simulink model "LINE_CONTROL"  (R2024a)
settings: Solver=ode4  StartTime=0.0  StopTime=10  FixedStep=1e-1  RelTol=1e-3
PreLoadFcn:
  | track_map = track_map;
values from neighbouring files (symbols this model uses):
  D_left = 1    [LINE_CONTROL_SETUP.m]    (also in x_opt.mat = 0.0771620798353)
  D_right = 1    [LINE_CONTROL_SETUP.m]    (also in x_opt.mat = 2.23648591389)
  I_left = 1    [LINE_CONTROL_SETUP.m]    (also in x_opt.mat = 1.054302631)
  I_right = 1    [LINE_CONTROL_SETUP.m]    (also in x_opt.mat = 1.261021045)
  L = 10e-2    (= 0.1)    [LINE_CONTROL_SETUP.m]    (also in x_opt.mat)
  P_left = 1    [LINE_CONTROL_SETUP.m]    (also in x_opt.mat = 2.23919550421)
  P_right = 1    [LINE_CONTROL_SETUP.m]    (also in x_opt.mat = 4.57741332247)
  r = 3.5e-2    (= 0.035)    [LINE_CONTROL_SETUP.m]    (also in x_opt.mat)
  theta_0 = deg2rad(0)    [LINE_CONTROL_SETUP.m]    (also in x_opt.mat = 0)
  x0 = 1    [LINE_CONTROL_SETUP.m]    (also in x_opt.mat)
  y0 = 1.146    [LINE_CONTROL_SETUP.m]    (also in x_opt.mat)
undefined symbols (not defined in the file or in its folder): k_1, k_2, k_3
libraries: slpidlib x2
settings Model: ParamWorkspaceSource=ReferencedWorkspace  Creator=pedro  LastModifiedBy=pedro

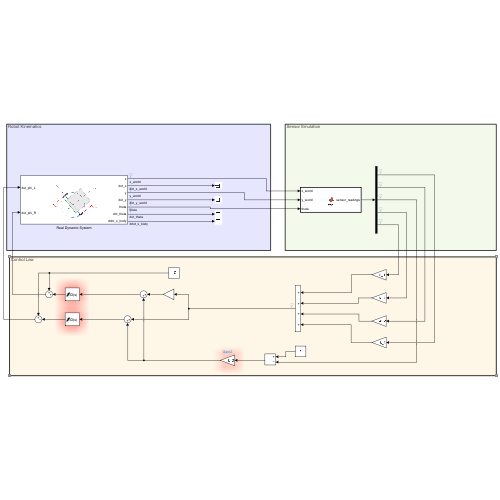
[thumbnail: Simulink's stored preview of the top-level diagram]
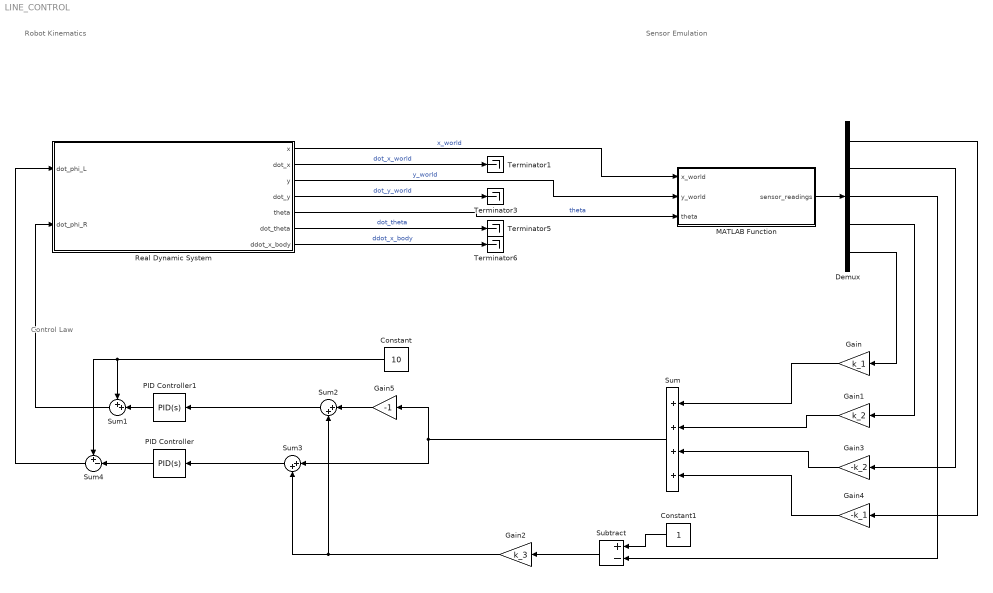
== system LINE_CONTROL ==
  note: Control Law
  note: Sensor Emulation
  note: Robot Kinematics
  Constant : Constant  Value=10
  Constant1 : Constant
  Demux : Demux  Outputs=5
  Gain : Gain  Gain=k_1
  Gain1 : Gain  Gain=k_2
  Gain2 : Gain  Gain=k_3
  Gain3 : Gain  Gain=-k_2
  Gain4 : Gain  Gain=-k_1
  Gain5 : Gain  Gain=-1
  MATLAB Function : MATLAB Function  TreatAsAtomicUnit=on
  PID Controller : slpidlib/PID Controller  Controller=PID  Form=Ideal  TimeDomain=Continuous-time  UseExternalTs=off  SampleTime=-1  IntegratorMethod=Forward Euler  FilterMethod=Forward Euler  ControllerParametersSource=internal  P=P_left  I=I_left  UseKiTs=off  D=D_left  UseExternalDerivativeSource=off  N=100  UseFilter=on  TunerSelectOption=Transfer Function Based (PID Tuner App)  InitialConditionSource=internal  InitialConditionForIntegrator=0  InitialConditionForFilter=0  DifferentiatorICPrevScaledInput=0  ExternalReset=none  TrackingMode=off  Kt=1  LimitOutput=on  SatLimitsSource=internal  UpperSaturationLimit=20  LowerSaturationLimit=-20  LinearizeAsGain=on  AntiWindupMode=clamping  Kb=1  LimitIntegrator=off  UpperIntegratorSaturationLimit=inf  LowerIntegratorSaturationLimit=-inf  POutMin=[]  POutMax=[]  IOutMin=[]  IOutMax=[]  DOutMin=[]  DOutMax=[]  NOutMin=[]  NOutMax=[]  SumOutMin=[]  SumOutMax=[]  SaturationOutMin=[]  SaturationOutMax=[]  PParamMin=[]  PParamMax=[]  IParamMin=[]  IParamMax=[]  DParamMin=[]  DParamMax=[]  NParamMin=[]  NParamMax=[]  KbParamMin=[]  KbParamMax=[]  KtParamMin=[]  KtParamMax=[]  KbOutMin=[]  KbOutMax=[]  KtOutMin=[]  KtOutMax=[]  IntegratorOutMin=[]  IntegratorOutMax=[]  FilterOutMin=[]  FilterOutMax=[]  SumI1OutMin=[]  SumI1OutMax=[]  SumI2OutMin=[]  SumI2OutMax=[]  SumI3OutMin=[]  SumI3OutMax=[]  SumI4OutMin=[]  SumI4OutMax=[]  SumDOutMin=[]  SumDOutMax=[]  DifferentiatorOutMin=[]  DifferentiatorOutMax=[]  FilterDiffOutCoefMin=[]  FilterDiffOutCoefMax=[]  ReciprocalOutMin=[]  ReciprocalOutMax=[]  SumDenOutMin=[]  SumDenOutMax=[]  SumNumOutMin=[]  SumNumOutMax=[]  DivideOutMin=[]  DivideOutMax=[]  UdiffTsProdOutMin=[]  UdiffTsProdOutMax=[]  NTsProdOutMin=[]  NTsProdOutMax=[]  UintegralTsProdOutMin=[]  UintegralTsProdOutMax=[]  UngainTsProdOutMin=[]  UngainTsProdOutMax=[]  ClampingZeroOutDataTypeStr=Inherit: Inherit via back propagation  ClampingZeroOutMin=[]  ClampingZeroOutMax=[]  FilterDenConstantOutDataTypeStr=Inherit: Inherit via back propagation  FilterDenConstantOutMin=[]  FilterDenConstantOutMax=[]  PCopyOutDataTypeStr=Inherit: Inherit via back propagation  PCopyOutMin=[]  PCopyOutMax=[]  NCopyOutDataTypeStr=Inherit: Inherit via back propagation  NCopyOutMin=[]  NCopyOutMax=[]  IntegratorContinuousStateAttributes=''  IntegratorStateMustResolveToSignalObject=off  IntegratorRTWStateStorageClass=Auto  FilterContinuousStateAttributes=''  FilterStateMustResolveToSignalObject=off  FilterRTWStateStorageClass=Auto  ParallelPVariant=Passthrough  IdealPVariant=InternalParameters  IVariant=InternalParameters  DVariant=InternalParameters  IntegratorVariant=Continuous  SatVariant=Enabled  AWVariant=ContClampingIdeal  PCopyVariant=InternalParamsIdeal  TRVariant=Disabled  FdbkBlocksVariant=Forward  IdealPFdbkVariant=Disabled  SatFdbkVariant=Disabled  DerivativeFilterVariant=ContFilter  NVariant=InternalParameters  NCopyVariant=Disabled  FilterICVariant=InternalICsFilter  IntegratorICVariant=InternalICs  ExternalResetVariant=Disabled  TRSumVariant=Passthrough  SumFdbkVariant=Disabled  SumVariant=Sum_PID  TsampFilterVariant=InternalTs  TsampNgainVariant=Passthrough  TsampIntegralVariant=Disabled_SignalSpec  ExternalSaturationOutDataTypeStr=Inherit: Same as second input  DerivativeSourceVariant=ErrorSignal
  PID Controller1 : slpidlib/PID Controller  Controller=PID  Form=Ideal  TimeDomain=Continuous-time  UseExternalTs=off  SampleTime=-1  IntegratorMethod=Forward Euler  FilterMethod=Forward Euler  ControllerParametersSource=internal  P=P_right  I=I_right  UseKiTs=off  D=D_right  UseExternalDerivativeSource=off  N=100  UseFilter=on  TunerSelectOption=Transfer Function Based (PID Tuner App)  InitialConditionSource=internal  InitialConditionForIntegrator=0  InitialConditionForFilter=0  DifferentiatorICPrevScaledInput=0  ExternalReset=none  TrackingMode=off  Kt=1  LimitOutput=on  SatLimitsSource=internal  UpperSaturationLimit=20  LowerSaturationLimit=-20  LinearizeAsGain=on  AntiWindupMode=clamping  Kb=1  LimitIntegrator=off  UpperIntegratorSaturationLimit=inf  LowerIntegratorSaturationLimit=-inf  POutMin=[]  POutMax=[]  IOutMin=[]  IOutMax=[]  DOutMin=[]  DOutMax=[]  NOutMin=[]  NOutMax=[]  SumOutMin=[]  SumOutMax=[]  SaturationOutMin=[]  SaturationOutMax=[]  PParamMin=[]  PParamMax=[]  IParamMin=[]  IParamMax=[]  DParamMin=[]  DParamMax=[]  NParamMin=[]  NParamMax=[]  KbParamMin=[]  KbParamMax=[]  KtParamMin=[]  KtParamMax=[]  KbOutMin=[]  KbOutMax=[]  KtOutMin=[]  KtOutMax=[]  IntegratorOutMin=[]  IntegratorOutMax=[]  FilterOutMin=[]  FilterOutMax=[]  SumI1OutMin=[]  SumI1OutMax=[]  SumI2OutMin=[]  SumI2OutMax=[]  SumI3OutMin=[]  SumI3OutMax=[]  SumI4OutMin=[]  SumI4OutMax=[]  SumDOutMin=[]  SumDOutMax=[]  DifferentiatorOutMin=[]  DifferentiatorOutMax=[]  FilterDiffOutCoefMin=[]  FilterDiffOutCoefMax=[]  ReciprocalOutMin=[]  ReciprocalOutMax=[]  SumDenOutMin=[]  SumDenOutMax=[]  SumNumOutMin=[]  SumNumOutMax=[]  DivideOutMin=[]  DivideOutMax=[]  UdiffTsProdOutMin=[]  UdiffTsProdOutMax=[]  NTsProdOutMin=[]  NTsProdOutMax=[]  UintegralTsProdOutMin=[]  UintegralTsProdOutMax=[]  UngainTsProdOutMin=[]  UngainTsProdOutMax=[]  ClampingZeroOutDataTypeStr=Inherit: Inherit via back propagation  ClampingZeroOutMin=[]  ClampingZeroOutMax=[]  FilterDenConstantOutDataTypeStr=Inherit: Inherit via back propagation  FilterDenConstantOutMin=[]  FilterDenConstantOutMax=[]  PCopyOutDataTypeStr=Inherit: Inherit via back propagation  PCopyOutMin=[]  PCopyOutMax=[]  NCopyOutDataTypeStr=Inherit: Inherit via back propagation  NCopyOutMin=[]  NCopyOutMax=[]  IntegratorContinuousStateAttributes=''  IntegratorStateMustResolveToSignalObject=off  IntegratorRTWStateStorageClass=Auto  FilterContinuousStateAttributes=''  FilterStateMustResolveToSignalObject=off  FilterRTWStateStorageClass=Auto  ParallelPVariant=Passthrough  IdealPVariant=InternalParameters  IVariant=InternalParameters  DVariant=InternalParameters  IntegratorVariant=Continuous  SatVariant=Enabled  AWVariant=ContClampingIdeal  PCopyVariant=InternalParamsIdeal  TRVariant=Disabled  FdbkBlocksVariant=Forward  IdealPFdbkVariant=Disabled  SatFdbkVariant=Disabled  DerivativeFilterVariant=ContFilter  NVariant=InternalParameters  NCopyVariant=Disabled  FilterICVariant=InternalICsFilter  IntegratorICVariant=InternalICs  ExternalResetVariant=Disabled  TRSumVariant=Passthrough  SumFdbkVariant=Disabled  SumVariant=Sum_PID  TsampFilterVariant=InternalTs  TsampNgainVariant=Passthrough  TsampIntegralVariant=Disabled_SignalSpec  ExternalSaturationOutDataTypeStr=Inherit: Same as second input  DerivativeSourceVariant=ErrorSignal
  Real Dynamic System : Subsystem
      mask Display: image('robot_model.png', [0,0,0,0,90,90]);
  Subtract : Sum  Inputs=+-
  Sum : Sum  Inputs=++++
  Sum1 : Sum  Inputs=++|
  Sum2 : Sum  Inputs=|++
  Sum3 : Sum  Inputs=|++
  Sum4 : Sum  Inputs=+-|
  Terminator{1,3,5..6} (4 alike) : Terminator
  wires:
  Real Dynamic System/1(x) -> MATLAB Function/1(x_world)  "x_world"
  Real Dynamic System/2(dot_x) -> Terminator1/1  "dot_x_world"
  Real Dynamic System/3(y) -> MATLAB Function/2(y_world)  "y_world"
  Real Dynamic System/4(dot_y) -> Terminator3/1  "dot_y_world"
  Real Dynamic System/5(theta) -> MATLAB Function/3(theta)  "theta"
  Real Dynamic System/6(dot_theta) -> Terminator5/1  "dot_theta"
  Real Dynamic System/7(ddot_x_body) -> Terminator6/1  "ddot_x_body"
  MATLAB Function/1(sensor_readings) -> Demux/1
  Demux/5 -> Gain/1
  Demux/4 -> Gain1/1
  Demux/3 -> Subtract/2
  Demux/2 -> Gain3/1
  Demux/1 -> Gain4/1
  Gain/1 -> Sum/1
  Gain1/1 -> Sum/2
  Gain3/1 -> Sum/3
  Gain4/1 -> Sum/4
  Constant/1 -> Sum4/1, Sum1/1
  Sum/1 -> Sum3/1, Gain5/1
  Gain5/1 -> Sum2/1
  Sum2/1 -> PID Controller1/1
  PID Controller1/1 -> Sum1/2
  Sum1/1 -> Real Dynamic System/2(dot_phi_R)
  PID Controller/1 -> Sum4/2
  Sum3/1 -> PID Controller/1
  Sum4/1 -> Real Dynamic System/1(dot_phi_L)
  Constant1/1 -> Subtract/1
  Subtract/1 -> Gain2/1
  Gain2/1 -> Sum2/2, Sum3/2

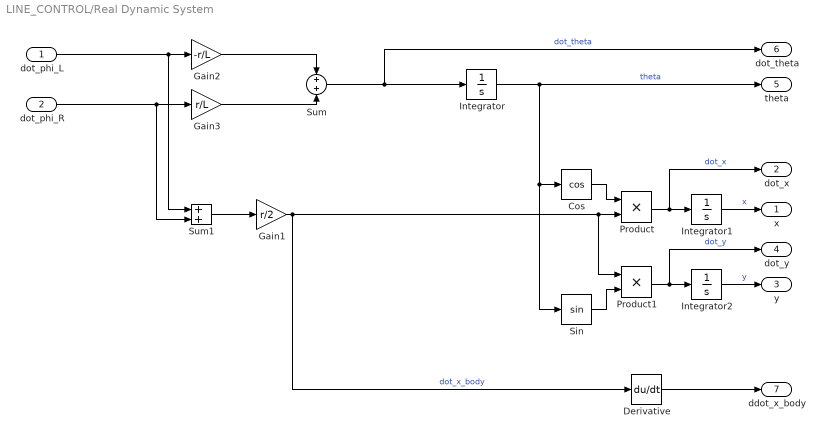
== system LINE_CONTROL/Real Dynamic System ==
  dot_phi_L : Inport
  dot_phi_R : Inport  Port=2
  Cos : Trigonometry  Operator=cos
  Derivative : Derivative
  Gain1 : Gain  Gain=r/2
  Gain2 : Gain  Gain=-r/L
  Gain3 : Gain  Gain=r/L
  Integrator : Integrator  InitialCondition=theta_0
  Integrator1 : Integrator  InitialCondition=x0
  Integrator2 : Integrator  InitialCondition=y0
  Product : Product
  Product1 : Product
  Sin : Trigonometry
  Sum : Sum  Inputs=+|+
  Sum1 : Sum
  x : Outport
  dot_x : Outport  Port=2
  y : Outport  Port=3
  dot_y : Outport  Port=4
  theta : Outport  Port=5
  dot_theta : Outport  Port=6
  ddot_x_body : Outport  Port=7
  wires:
  dot_phi_L/1 -> Sum1/1, Gain2/1
  Product1/1 -> dot_y/1, Integrator2/1  "dot_y"
  Cos/1 -> Product/1
  Integrator/1 -> theta/1, Sin/1, Cos/1  "theta"
  Gain3/1 -> Sum/2
  Product/1 -> dot_x/1, Integrator1/1  "dot_x"
  Gain1/1 -> Derivative/1, Product1/1, Product/2  "dot_x_body"
  Sum1/1 -> Gain1/1
  dot_phi_R/1 -> Sum1/2, Gain3/1
  Gain2/1 -> Sum/1
  Sum/1 -> dot_theta/1, Integrator/1  "dot_theta"
  Integrator1/1 -> x/1  "x"
  Integrator2/1 -> y/1  "y"
  Sin/1 -> Product1/2
  Derivative/1 -> ddot_x_body/1

== matlab function LINE_CONTROL/MATLAB Function ==
  data: x_world input; sensor_readings output; y_world input; theta input; track_map parameter
function sensor_readings = fcn(x_world, y_world, theta, track_map)


rotation_matrix = [cos(theta) -sin(theta)
                    sin(theta) cos(theta)];

x_world = squeeze(x_world);
y_world = squeeze(y_world);
theta   = squeeze(theta);

P_sensor_1 = [5.5e-2  7e-2]';
P_sensor_2 = [3e-2    7e-2]';
P_sensor_3 = [0     8.5e-2]';
P_sensor_4 = [-3e-2   7e-2]';
P_sensor_5 = [-5.5e-2 7e-2]';

sensor_1_coord = [x_world y_world]' + rotation_matrix * P_sensor_1;
sensor_2_coord = [x_world y_world]' + rotation_matrix * P_sensor_2;
sensor_3_coord = [x_world y_world]' + rotation_matrix * P_sensor_3;
sensor_4_coord = [x_world y_world]' + rotation_matrix * P_sensor_4;
sensor_5_coord = [x_world y_world]' + rotation_matrix * P_sensor_5;

sensor_1_coord = ceil(sensor_1_coord*1e3); % Convert to mm since 1px=1mm
sensor_2_coord = ceil(sensor_2_coord*1e3); % Convert to mm since 1px=1mm
sensor_3_coord = ceil(sensor_3_coord*1e3); % Convert to mm since 1px=1mm
sensor_4_coord = ceil(sensor_4_coord*1e3); % Convert to mm since 1px=1mm
sensor_5_coord = ceil(sensor_5_coord*1e3); % Convert to mm since 1px=1mm

%max_line_sensor_value = 2500;
%min_line_sensor_value = 500;

track_index_size = flip(size(track_map));
sensor_readings = zeros(1, 5);

if any(track_index_size' < [sensor_1_coord sensor_2_coord sensor_3_coord sensor_4_coord sensor_5_coord], 'all') || any([0;0] >= [sensor_1_coord sensor_2_coord sensor_3_coord sensor_4_coord sensor_5_coord], 'all')
    %sensor_readings(sensor_readings == 0) = min_line_sensor_value;
    return
end

sensor_readings(1) = track_map(sensor_1_coord(2), sensor_1_coord(1));
sensor_readings(2) = track_map(sensor_2_coord(2), sensor_2_coord(1));
sensor_readings(3) = track_map(sensor_3_coord(2), sensor_3_coord(1));
sensor_readings(4) = track_map(sensor_4_coord(2), sensor_4_coord(1));
sensor_readings(5) = track_map(sensor_5_coord(2), sensor_5_coord(1));

%sensor_readings(sensor_readings == 0)   = min_line_sensor_value;
%sensor_readings(sensor_readings == 1) = max_line_sensor_value;
